simulink model "TestKit2"  (R2024b)
settings: Solver=FixedStepAuto  StartTime=0.0  StopTime=inf  FixedStep=0.1  RelTol=1e-3  EnableMultiTasking=on
libraries: stm32f4xxblockslib x8, stm32g4xxblockslib x6
settings Model: STM32="{\"EncoderBlockForG4\":[{\"ID\":\"TestKit2:1\"},{\"ID\":\"TestKit2:5\"},{\"ID\":\"TestKit2:7\"},{\"ID\":\"TestKit2:156\"},{\"ID\":\"TestKit2:157\"},{\"ID\":\"TestKit2:158\"}],\"DigitalPortRead\":[{\"ID\":\"TestKit2:112\"},{\"ID\":\"TestKit2:64\"},{\"ID\":\"TestKit2:65\"},{\"ID\":\"TestKit2:111\"},{\"ID\":\"TestKit2:128\"},{\"ID\":\"TestKit2:129\"},{\"ID\":\"TestKit2:130\"},{\"ID\":\"TestKit2:131\"}]}"  SimulationMode=external  Creator=KritZ  LastModifiedBy=KritZ
settings OptimizationCC: DefaultParameterBehavior=Inlined  EnhancedBackFolding=on  PassReuseOutputArgsAs=Individual arguments  ZeroExternalMemoryAtStartup=off  ZeroInternalMemoryAtStartup=off  MaxStackSize=512  OptimizeBlockOrder=speed  DifferentSizesBufferReuse=on  OptimizationCustomize=off  EfficientTunableParamExpr=on
settings DebuggingCC: ParameterTunabilityLossMsg=error
settings HardwareCC: ProdBitPerPointer=32  ProdBitPerSizeT=32  ProdBitPerPtrDiffT=32  ProdLargestAtomicInteger=Long  ProdLargestAtomicFloat=Double  ProdWordSize=32  ProdLongLongMode=on  ProdHWDeviceType=ARM Compatible->ARM Cortex-M
settings SFSimCC: MATLABDynamicMemAlloc=off
settings RTWCC: Description=Embedded Coder  SystemTargetFile=ert.tlc  HardwareBoard=STM32G4xx Based  TemplateMakefile=ert_default_tmf  Toolchain=GNU Tools for ARM Embedded Processors
settings CodeAppCC: ForceParamTrailComments=on  IgnoreCustomStorageClasses=off  OperatorAnnotations=on  SimulinkDataObjDesc=on  SFDataObjDesc=on  InsertBlockDesc=on
settings ERTTargetCC: TargetLangStandard=C99 (ISO)  CodeReplacementLibrary=ARM Cortex-M  SupportContinuousTime=on  ExtModeTransport=3  ExtModeStaticAlloc=on  ExtModeStaticAllocSize=2048  ExtModeMexFile=ext_xcp  ExtModeIntrfLevel=Level2 - Open

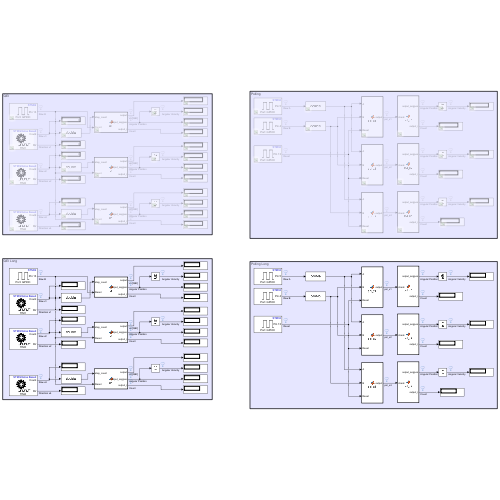
[thumbnail: Simulink's stored preview of the top-level diagram]
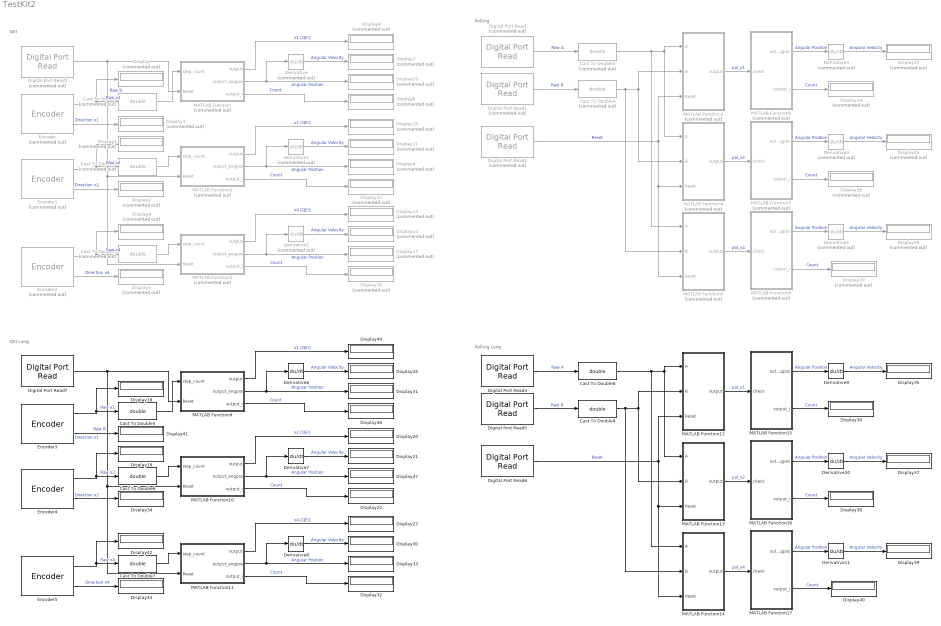
== system TestKit2 ==
  note: Polling
  note: QEI
  note: QEI Long
  note: Polling Long
  Cast To Double{,1..4} (5 alike) : DataTypeConversion  Commented=on  OutDataTypeStr=double  SaturateOnIntegerOverflow=off  RndMeth=Floor
  Cast To Double{5..9} (5 alike) : DataTypeConversion  OutDataTypeStr=double  SaturateOnIntegerOverflow=off  RndMeth=Floor
  Derivative{,1..5} (6 alike) : Derivative  Commented=on
  Derivative{6..11} (6 alike) : Derivative
  Digital Port Read : stm32f4xxblockslib/Digital Port Read  Commented=on  PortName=GPIOC  PinNumber=5  ReadOperation=on  IOAsArray=off  SampleTime=-1  EnableSimPort=off  hoistedMaskSrc=ECSoC/ECSimCodegen/Digital Port Read
      settings: LibrarySourceBlock=stm32g4xxblockslib/Digital Port Read
  Digital Port Read1 : stm32f4xxblockslib/Digital Port Read  Commented=on  PortName=GPIOC  PinNumber=4  ReadOperation=on  IOAsArray=off  SampleTime=-1  EnableSimPort=off  hoistedMaskSrc=ECSoC/ECSimCodegen/Digital Port Read
      settings: LibrarySourceBlock=stm32g4xxblockslib/Digital Port Read
  Digital Port Read2 : stm32f4xxblockslib/Digital Port Read  Commented=on  PortName=GPIOC  PinNumber=13  ReadOperation=on  IOAsArray=off  SampleTime=-1  EnableSimPort=off  hoistedMaskSrc=ECSoC/ECSimCodegen/Digital Port Read
      settings: LibrarySourceBlock=stm32g4xxblockslib/Digital Port Read
  Digital Port Read3 : stm32f4xxblockslib/Digital Port Read  Commented=on  PortName=GPIOC  PinNumber=13  ReadOperation=on  IOAsArray=off  SampleTime=-1  EnableSimPort=off  hoistedMaskSrc=ECSoC/ECSimCodegen/Digital Port Read
      settings: LibrarySourceBlock=stm32g4xxblockslib/Digital Port Read
  Digital Port Read4 : stm32f4xxblockslib/Digital Port Read  PortName=GPIOC  PinNumber=5  ReadOperation=on  IOAsArray=off  SampleTime=-1  EnableSimPort=off  hoistedMaskSrc=ECSoC/ECSimCodegen/Digital Port Read
      settings: LibrarySourceBlock=stm32g4xxblockslib/Digital Port Read
  Digital Port Read5 : stm32f4xxblockslib/Digital Port Read  PortName=GPIOC  PinNumber=4  ReadOperation=on  IOAsArray=off  SampleTime=-1  EnableSimPort=off  hoistedMaskSrc=ECSoC/ECSimCodegen/Digital Port Read
      settings: LibrarySourceBlock=stm32g4xxblockslib/Digital Port Read
  Digital Port Read6 : stm32f4xxblockslib/Digital Port Read  PortName=GPIOC  PinNumber=13  ReadOperation=on  IOAsArray=off  SampleTime=-1  EnableSimPort=off  hoistedMaskSrc=ECSoC/ECSimCodegen/Digital Port Read
      settings: LibrarySourceBlock=stm32g4xxblockslib/Digital Port Read
  Digital Port Read7 : stm32f4xxblockslib/Digital Port Read  PortName=GPIOC  PinNumber=13  ReadOperation=on  IOAsArray=off  SampleTime=-1  EnableSimPort=off  hoistedMaskSrc=ECSoC/ECSimCodegen/Digital Port Read
      settings: LibrarySourceBlock=stm32g4xxblockslib/Digital Port Read
  Display{,1..17,23..26,28..29} (24 alike) : Display  Commented=on
  Display{18..22,27,30..47} (24 alike) : Display
  Encoder : stm32g4xxblockslib/Encoder  Commented=on  TimerModule=TIM1  EnableResetInput=off  OutputCountAfterFirstIndex=off  OutputValidIndex=off  OutputDirection=on  OutputStatus=off  SampleTime=-1
  Encoder1 : stm32g4xxblockslib/Encoder  Commented=on  TimerModule=TIM3  EnableResetInput=off  OutputCountAfterFirstIndex=off  OutputValidIndex=off  OutputDirection=on  OutputStatus=off  SampleTime=-1
  Encoder2 : stm32g4xxblockslib/Encoder  Commented=on  TimerModule=TIM4  EnableResetInput=off  OutputCountAfterFirstIndex=off  OutputValidIndex=off  OutputDirection=on  OutputStatus=off  SampleTime=-1
  Encoder3 : stm32g4xxblockslib/Encoder  TimerModule=TIM1  EnableResetInput=off  OutputCountAfterFirstIndex=off  OutputValidIndex=off  OutputDirection=on  OutputStatus=off  SampleTime=-1
  Encoder4 : stm32g4xxblockslib/Encoder  TimerModule=TIM3  EnableResetInput=off  OutputCountAfterFirstIndex=off  OutputValidIndex=off  OutputDirection=on  OutputStatus=off  SampleTime=-1
  Encoder5 : stm32g4xxblockslib/Encoder  TimerModule=TIM4  EnableResetInput=off  OutputCountAfterFirstIndex=off  OutputValidIndex=off  OutputDirection=on  OutputStatus=off  SampleTime=-1
  MATLAB Function : MATLAB Function  Commented=on  TreatAsAtomicUnit=on
  MATLAB Function1 : MATLAB Function  Commented=on  TreatAsAtomicUnit=on
  MATLAB Function10 : MATLAB Function  TreatAsAtomicUnit=on
  MATLAB Function11 : MATLAB Function  TreatAsAtomicUnit=on
  MATLAB Function12 : MATLAB Function  TreatAsAtomicUnit=on
  MATLAB Function13 : MATLAB Function  TreatAsAtomicUnit=on
  MATLAB Function14 : MATLAB Function  TreatAsAtomicUnit=on
  MATLAB Function15 : MATLAB Function  TreatAsAtomicUnit=on
  MATLAB Function16 : MATLAB Function  TreatAsAtomicUnit=on
  MATLAB Function17 : MATLAB Function  TreatAsAtomicUnit=on
  MATLAB Function2 : MATLAB Function  Commented=on  TreatAsAtomicUnit=on
  MATLAB Function3 : MATLAB Function  Commented=on  TreatAsAtomicUnit=on
  MATLAB Function4 : MATLAB Function  Commented=on  TreatAsAtomicUnit=on
  MATLAB Function5 : MATLAB Function  Commented=on  TreatAsAtomicUnit=on
  MATLAB Function6 : MATLAB Function  Commented=on  TreatAsAtomicUnit=on
  MATLAB Function7 : MATLAB Function  Commented=on  TreatAsAtomicUnit=on
  MATLAB Function8 : MATLAB Function  Commented=on  TreatAsAtomicUnit=on
  MATLAB Function9 : MATLAB Function  TreatAsAtomicUnit=on
  wires:
  Encoder/1 -> Display/1, Cast To Double/1  "Raw x1"
  Encoder/2 -> Display3/1  "Direction x1"
  Encoder1/2 -> Display2/1  "Direction x2"
  Encoder1/1 -> Display1/1, Cast To Double1/1  "Raw x2"
  Encoder2/1 -> Display4/1, Cast To Double2/1  "Raw x4"
  Encoder2/2 -> Display5/1  "Direction x4"
  Cast To Double/1 -> MATLAB Function/1(step_count)
  MATLAB Function/1(output) -> Display6/1  "x1 [QEI]"
  MATLAB Function/3(output_i) -> Display8/1  "Count"
  MATLAB Function/2(output_angpos) -> Display15/1, Derivative/1  "Angular Position"
  Digital Port Read/1 -> Cast To Double3/1  "Raw A"
  Digital Port Read1/1 -> Cast To Double4/1  "Raw B"
  Cast To Double3/1 -> MATLAB Function5/1(A), MATLAB Function4/1(A), MATLAB Function3/1(A)
  Cast To Double4/1 -> MATLAB Function5/2(B), MATLAB Function3/2(B), MATLAB Function4/2(B)
  MATLAB Function3/1(output) -> MATLAB Function6/1(check)  "pol_x1"
  MATLAB Function5/1(output) -> MATLAB Function8/1(check)  "pol_x4"
  Derivative/1 -> Display7/1  "Angular Velocity"
  Derivative1/1 -> Display11/1  "Angular Velocity"
  MATLAB Function1/2(output_angpos) -> Display9/1, Derivative1/1  "Angular Position"
  MATLAB Function1/3(output_i) -> Display12/1  "Count"
  MATLAB Function1/1(output) -> Display10/1  "x2 [QEI]"
  Cast To Double1/1 -> MATLAB Function1/1(step_count)
  MATLAB Function2/2(output_angpos) -> Display17/1, Derivative2/1  "Angular Position"
  MATLAB Function2/1(output) -> Display13/1  "x4 [QEI]"
  MATLAB Function2/3(output_i) -> Display16/1  "Count"
  Derivative2/1 -> Display14/1  "Angular Velocity"
  Cast To Double2/1 -> MATLAB Function2/1(step_count)
  MATLAB Function6/1(output_angpos) -> Derivative3/1  "Angular Position"
  Derivative3/1 -> Display23/1  "Angular Velocity"
  MATLAB Function6/2(output_i) -> Display24/1  "Count"
  MATLAB Function4/1(output) -> MATLAB Function7/1(check)  "pol_x2"
  MATLAB Function7/1(output_angpos) -> Derivative4/1  "Angular Position"
  Derivative4/1 -> Display25/1  "Angular Velocity"
  MATLAB Function8/1(output_angpos) -> Derivative5/1  "Angular Position"
  Derivative5/1 -> Display28/1  "Angular Velocity"
  MATLAB Function8/2(output_i) -> Display29/1  "Count"
  MATLAB Function7/2(output_i) -> Display26/1  "Count"
  Digital Port Read2/1 -> MATLAB Function5/3(Reset), MATLAB Function4/3(Reset), MATLAB Function3/3(Reset)  "Reset"
  Digital Port Read3/1 -> MATLAB Function2/2(Reset), MATLAB Function1/2(Reset), MATLAB Function/2(Reset)  "Raw B"
  Digital Port Read5/1 -> Cast To Double9/1  "Raw B"
  Derivative11/1 -> Display39/1  "Angular Velocity"
  Digital Port Read7/1 -> MATLAB Function11/2(Reset), MATLAB Function10/2(Reset), MATLAB Function9/2(Reset)  "Raw B"
  Encoder5/2 -> Display43/1  "Direction x4"
  Digital Port Read4/1 -> Cast To Double8/1  "Raw A"
  MATLAB Function16/1(output_angpos) -> Derivative10/1  "Angular Position"
  Encoder5/1 -> Display42/1, Cast To Double7/1  "Raw x4"
  Derivative9/1 -> Display35/1  "Angular Velocity"
  Cast To Double9/1 -> MATLAB Function14/2(B), MATLAB Function12/2(B), MATLAB Function13/2(B)
  Cast To Double8/1 -> MATLAB Function14/1(A), MATLAB Function13/1(A), MATLAB Function12/1(A)
  Cast To Double6/1 -> MATLAB Function10/1(step_count)
  MATLAB Function11/3(output_i) -> Display32/1  "Count"
  MATLAB Function17/2(output_i) -> Display40/1  "Count"
  Encoder3/2 -> Display41/1  "Direction x1"
  MATLAB Function9/3(output_i) -> Display46/1  "Count"
  MATLAB Function12/1(output) -> MATLAB Function15/1(check)  "pol_x1"
  Encoder3/1 -> Display18/1, Cast To Double5/1  "Raw x1"
  MATLAB Function14/1(output) -> MATLAB Function17/1(check)  "pol_x4"
  MATLAB Function16/2(output_i) -> Display38/1  "Count"
  Derivative6/1 -> Display45/1  "Angular Velocity"
  MATLAB Function11/2(output_angpos) -> Display33/1, Derivative8/1  "Angular Position"
  Cast To Double7/1 -> MATLAB Function11/1(step_count)
  MATLAB Function15/1(output_angpos) -> Derivative9/1  "Angular Position"
  MATLAB Function9/2(output_angpos) -> Display31/1, Derivative6/1  "Angular Position"
  Digital Port Read6/1 -> MATLAB Function14/3(Reset), MATLAB Function13/3(Reset), MATLAB Function12/3(Reset)  "Reset"
  MATLAB Function11/1(output) -> Display27/1  "x4 [QEI]"
  MATLAB Function10/3(output_i) -> Display22/1  "Count"
  MATLAB Function10/2(output_angpos) -> Display47/1, Derivative7/1  "Angular Position"
  MATLAB Function13/1(output) -> MATLAB Function16/1(check)  "pol_x2"
  Derivative10/1 -> Display37/1  "Angular Velocity"
  MATLAB Function17/1(output_angpos) -> Derivative11/1  "Angular Position"
  Derivative7/1 -> Display21/1  "Angular Velocity"
  Encoder4/1 -> Display19/1, Cast To Double6/1  "Raw x2"
  MATLAB Function15/2(output_i) -> Display36/1  "Count"
  MATLAB Function10/1(output) -> Display20/1  "x2 [QEI]"
  Encoder4/2 -> Display34/1  "Direction x2"
  Cast To Double5/1 -> MATLAB Function9/1(step_count)
  MATLAB Function9/1(output) -> Display44/1  "x1 [QEI]"
  Derivative8/1 -> Display30/1  "Angular Velocity"

== matlab function TestKit2/MATLAB Function11 ==
  data: output output; step_count input; output_angpos output; output_i output; Reset input
function [output,output_angpos,output_i] = x4(step_count,Reset)
    % Local variebles
    persistent check;
    persistent previous;
    persistent rev;
    persistent degree;


    % Check the reset button
    if Reset == 1
        check = 0;
    end
   

    % Initialize the state
    if isempty(check)
        check = 0; 
    end
    if isempty(previous)
        previous = 0;
    end
    if isempty(rev)
        rev = 0;
    end
    if isempty(degree)
        degree = 0;
    end

    % Distance between an old and a new one (to create a unlimit graph)
    getnumber = step_count - previous;
    if getnumber < -32760
        check = (check + (65520 + getnumber))+1;
    elseif getnumber > 32760
        check = (check - (65520 - getnumber))-1;
    else 
        check = check + getnumber;
    end

                                                                                            
    % Get a last data to print out
    previous = step_count;
    

    % Revolute & Degree
    rev = check / 2048;
    degree = rev*360;


    % Show a step time, velocity, unlimitted for encoder in rotate
    output = check;
    output_angpos = degree;
    output_i = rev; 
end


% function [output,output_angvelo,output_angpos,output_i] = x1(step_count)
%     % Local variebles
%     persistent next; 
%     persistent previous;
%     persistent i;
% 
% 
%     % Initialize the state
%     if isempty(next)
%         next = 0; 
%     end
%     if isempty(previous)
%         previous = 0;
%     end
%     if isempty(i)
%         i = 0;
%     end
% 
% 
%     % Distance between an old and a new one (to create a unlimit graph)
%     getnumber = step_count-previous;
%     if getnumber <= -32760
%         getnumber = 1;
%     elseif getnumber >= 32760
%         getnumber = -1;
%     end
% 
% 
%     % Get a last data to print out
%     next = getnumber+next;
%     previous = step_count;
% 
% 
%     % Angular & Velocity
%     velocity = getnumber/0.1;
%     omeaga = velocity/9.5;
% 
% 
%     % Zeta & Radians
%     zeta = omeaga * 0.1;
%     radian = (pi/180)*zeta;
% 
% 
%     % Show a step time, velocity, unlimitted for encoder in rotate
%     output = next;
%     output_angvelo = omeaga;
%     output_angpos = radian;
%     output_i = floor(abs(next/24)); 
% end
% 
% function [output,output_angvelo,output_angpos,output_i] = x1(step_count)
%     % Local variebles
%     persistent check;
%     persistent previous;
%     persistent i;
% 
% 
%     % Initialize the state
%     if isempty(check)
%         check = 0; 
%     end
%     if isempty(previous)
%         previous = 0;
%     end
%     if isempty(i)
%         i = 0;
%     end
% 
% 
%     % Distance between an old and a new one (to create a unlimit graph)
%     getnumber = step_count-previous;
%     if getnumber < -32760
%         check = (check - (65520-getnumber))+1;
%     elseif getnumber > 32760
%         check = (check - (65520+getnumber))-1;
%     else 
%         check = check+getnumber;
%     end
% 
% 
%     % Get a last data to print out
%     previous = step_count;
% 
% 
%     % Angular & Velocity
%     velocity = getnumber/0.1;
%     omeaga = velocity/9.5;
% 
% 
%     % Zeta & Radians
%     zeta = omeaga * 0.1;
%     radian = (pi/180)*zeta;
% 
% 
%     % Show a step time, velocity, unlimitted for encoder in rotate
%     output = check;
%     output_angvelo = omeaga;
%     output_angpos = radian;
%     output_i = floor(abs(check/24)); 
% end

== matlab function TestKit2/MATLAB Function12 ==
  data: A input; output output; B input; Reset input
function output = pol_x1(A,B,Reset)
    % Identifly a variable
    persistent count; 
    persistent previous;
    

    % Check the reset button
    if Reset == 1
        count = 0;
    end

    
    % Initialize the state on the first call
    if isempty(count)
        count = 0;
    end
    if isempty(previous)
        previous = 0;
    end
    

    % Condition for x1 [clockwise and counter-clockwise]
    if A == 1 && previous == 0
        if A == 1 && B == 0
            count = count + 1;
        elseif A == 1 && B == 1
            count = count - 1;
        end
    end


    % Get a last data to print out
    previous = A;


    % Output
    output = count;

== matlab function TestKit2/MATLAB Function1 ==
  data: output output; step_count input; output_angpos output; output_i output; Reset input
function [output,output_angpos,output_i] = x2(step_count,Reset)
    % Local variebles
    persistent check;
    persistent previous;
    persistent rev;
    persistent degree;


    % Check the reset button
    if Reset == 1
        check = 0;
    end
   

    % Initialize the state
    if isempty(check)
        check = 0; 
    end
    if isempty(previous)
        previous = 0;
    end
    if isempty(rev)
        rev = 0;
    end
    if isempty(degree)
        degree = 0;
    end

    % Distance between an old and a new one (to create a unlimit graph)
    getnumber = step_count - previous;
    if getnumber < -32760
        check = (check + (65520 + getnumber))+1;
    elseif getnumber > 32760
        check = (check - (65520 - getnumber))-1;
    else 
        check = check + getnumber;
    end

                                                                                            
    % Get a last data to print out
    previous = step_count;
    

    % Revolute & Degree
    rev = check / 24;
    degree = rev*360;


    % Show a step time, velocity, unlimitted for encoder in rotate
    output = check;
    output_angpos = degree;
    output_i = rev; 
end


% function [output,output_angvelo,output_angpos,output_i] = x1(step_count)
%     % Local variebles
%     persistent next; 
%     persistent previous;
%     persistent i;
% 
% 
%     % Initialize the state
%     if isempty(next)
%         next = 0; 
%     end
%     if isempty(previous)
%         previous = 0;
%     end
%     if isempty(i)
%         i = 0;
%     end
% 
% 
%     % Distance between an old and a new one (to create a unlimit graph)
%     getnumber = step_count-previous;
%     if getnumber <= -32760
%         getnumber = 1;
%     elseif getnumber >= 32760
%         getnumber = -1;
%     end
% 
% 
%     % Get a last data to print out
%     next = getnumber+next;
%     previous = step_count;
% 
% 
%     % Angular & Velocity
%     velocity = getnumber/0.1;
%     omeaga = velocity/9.5;
% 
% 
%     % Zeta & Radians
%     zeta = omeaga * 0.1;
%     radian = (pi/180)*zeta;
% 
% 
%     % Show a step time, velocity, unlimitted for encoder in rotate
%     output = next;
%     output_angvelo = omeaga;
%     output_angpos = radian;
%     output_i = floor(abs(next/24)); 
% end
% 
% function [output,output_angvelo,output_angpos,output_i] = x1(step_count)
%     % Local variebles
%     persistent check;
%     persistent previous;
%     persistent i;
% 
% 
%     % Initialize the state
%     if isempty(check)
%         check = 0; 
%     end
%     if isempty(previous)
%         previous = 0;
%     end
%     if isempty(i)
%         i = 0;
%     end
% 
% 
%     % Distance between an old and a new one (to create a unlimit graph)
%     getnumber = step_count-previous;
%     if getnumber < -32760
%         check = (check - (65520-getnumber))+1;
%     elseif getnumber > 32760
%         check = (check - (65520+getnumber))-1;
%     else 
%         check = check+getnumber;
%     end
% 
% 
%     % Get a last data to print out
%     previous = step_count;
% 
% 
%     % Angular & Velocity
%     velocity = getnumber/0.1;
%     omeaga = velocity/9.5;
% 
% 
%     % Zeta & Radians
%     zeta = omeaga * 0.1;
%     radian = (pi/180)*zeta;
% 
% 
%     % Show a step time, velocity, unlimitted for encoder in rotate
%     output = check;
%     output_angvelo = omeaga;
%     output_angpos = radian;
%     output_i = floor(abs(check/24)); 
% end

== matlab function TestKit2/MATLAB Function13 ==
  data: A input; output output; B input; Reset input
function output = pol_x2(A,B,Reset)
    % Identifly a variable
    persistent count; 
    persistent previous;
    

    % Check the reset button
    if Reset == 1
        count = 0;
    end


    % Initialize the state on the first call
    if isempty(count)
        count = 0;
    end
    if isempty(previous)
        previous = 0;
    end
    

    % Condition for x2 [clockwise and counter-clockwise]
    if A == 1 && previous == 0
        if A == 1 && B == 0
            count = count + 1;
        elseif A == 0 && B == 1
            count = count + 1;
        elseif A == 1 && B == 1
            count = count - 1;
        elseif A == 0 && B == 0
            count = count - 1;
        end 
    elseif A == 0 && previous == 1
        if A == 1 && B == 0
            count = count + 1;
        elseif A == 0 && B == 1
            count = count + 1;
        elseif A == 1 && B == 1
            count = count - 1;
        elseif A == 0 && B == 0
            count = count - 1;
        end  
    end


    % Get a last data to print out
    previous = A;


    % Output
    output = count;

== matlab function TestKit2/MATLAB Function14 ==
  data: A input; output output; B input; Reset input
function output = pol_x4(A,B,Reset)
    % Identifly a variable
    persistent count; 
    persistent previous_A;
    persistent previous_B;


    % Check the reset button
    if Reset == 1
        count = 0;
    end


    % Initialize the state on the first call
    if isempty(count)
        count = 0;
    end
    if isempty(previous_A)
        previous_A = 0;
    end
    if isempty(previous_B)
        previous_B = 0;
    end


    % Condition for x4A & x4B [clockwise and counter-clockwise]
    if A == 1 && previous_A == 0
        if B == 0
            count = count + 1;
        else 
            count = count - 1;
        end
    elseif A == 0 && previous_A == 1 
        if B == 1
            count = count + 1;
        else 
            count = count - 1;
        end
    elseif B == 1 && previous_B == 0
        if A == 1
            count = count + 1;
        else 
            count = count - 1;
        end
    elseif B == 0 && previous_B == 1 
        if A == 0
            count = count + 1;
        else
            count = count - 1;
        end
    end


    % Get a last data to print out
    previous_A = A;
    previous_B = B;


    % Output
    output = count;

== matlab function TestKit2/MATLAB Function15 ==
  data: check input; output_angpos output; output_i output
function [output_angpos,output_i] = out_x1(check)
    % Identifly a variable
    persistent count;


    % Initialize the state on the first call
    if isempty(count)
        count = 0;
    end


    % Revolute & Degree
    rev = check / 2048;
    degree = rev*360;
    radian = degree*2*pi;


    % Show a step time, velocity for encoder in rotate
    output_angpos = radian;
    output_i = rev;

== matlab function TestKit2/MATLAB Function16 ==
  data: check input; output_angpos output; output_i output
function [output_angpos,output_i] = out_x2(check)
    % Identifly a variable
    persistent count;


    % Initialize the state on the first call
    if isempty(count)
        count = 0;
    end


    % Revolute & Degree
    rev = check / (2048*2);
    degree = rev*360;
    radian = degree*2*pi;


    % Show a step time, velocity for encoder in rotate
    output_angpos = radian;
    output_i = rev;

== matlab function TestKit2/MATLAB Function17 ==
  data: check input; output_angpos output; output_i output
function [output_angpos,output_i] = out_x4(check)
    % Identifly a variable
    persistent count;


    % Initialize the state on the first call
    if isempty(count)
        count = 0;
    end


    % Revolute & Degree
    rev = check / (2048*4);
    degree = rev*360;
    radian = degree*2*pi;


    % Show a step time, velocity for encoder in rotate
    output_angpos = radian;
    output_i = rev;

== matlab function TestKit2/MATLAB Function9 ==
  data: output output; step_count input; output_angpos output; output_i output; Reset input
function [output,output_angpos,output_i] = x1(step_count,Reset)
    % Local variebles
    persistent check;
    persistent previous;
    persistent rev;
    persistent degree;


    % Check the reset button
    if Reset == 1
        check = 0;
    end
   

    % Initialize the state
    if isempty(check)
        check = 0; 
    end
    if isempty(previous)
        previous = 0;
    end
    if isempty(rev)
        rev = 0;
    end
    if isempty(degree)
        degree = 0;
    end

    % Distance between an old and a new one (to create a unlimit graph)
    getnumber = step_count - previous;
    if getnumber < -32760
        check = (check + (65520 + getnumber))+1;
    elseif getnumber > 32760
        check = (check - (65520 - getnumber))-1;
    else 
        check = check + getnumber;
    end

                                                                                            
    % Get a last data to print out
    previous = step_count;
    

    % Revolute & Degree
    rev = check / 2048;
    degree = rev*360;


    % Show a step time, velocity, unlimitted for encoder in rotate
    output = check;
    output_angpos = degree;
    output_i = rev; 
end


% function [output,output_angvelo,output_angpos,output_i] = x1(step_count)
%     % Local variebles
%     persistent next; 
%     persistent previous;
%     persistent i;
% 
% 
%     % Initialize the state
%     if isempty(next)
%         next = 0; 
%     end
%     if isempty(previous)
%         previous = 0;
%     end
%     if isempty(i)
%         i = 0;
%     end
% 
% 
%     % Distance between an old and a new one (to create a unlimit graph)
%     getnumber = step_count-previous;
%     if getnumber <= -32760
%         getnumber = 1;
%     elseif getnumber >= 32760
%         getnumber = -1;
%     end
% 
% 
%     % Get a last data to print out
%     next = getnumber+next;
%     previous = step_count;
% 
% 
%     % Angular & Velocity
%     velocity = getnumber/0.1;
%     omeaga = velocity/9.5;
% 
% 
%     % Zeta & Radians
%     zeta = omeaga * 0.1;
%     radian = (pi/180)*zeta;
% 
% 
%     % Show a step time, velocity, unlimitted for encoder in rotate
%     output = next;
%     output_angvelo = omeaga;
%     output_angpos = radian;
%     output_i = floor(abs(next/24)); 
% end
% 
% function [output,output_angvelo,output_angpos,output_i] = x1(step_count)
%     % Local variebles
%     persistent check;
%     persistent previous;
%     persistent i;
% 
% 
%     % Initialize the state
%     if isempty(check)
%         check = 0; 
%     end
%     if isempty(previous)
%         previous = 0;
%     end
%     if isempty(i)
%         i = 0;
%     end
% 
% 
%     % Distance between an old and a new one (to create a unlimit graph)
%     getnumber = step_count-previous;
%     if getnumber < -32760
%         check = (check - (65520-getnumber))+1;
%     elseif getnumber > 32760
%         check = (check - (65520+getnumber))-1;
%     else 
%         check = check+getnumber;
%     end
% 
% 
%     % Get a last data to print out
%     previous = step_count;
% 
% 
%     % Angular & Velocity
%     velocity = getnumber/0.1;
%     omeaga = velocity/9.5;
% 
% 
%     % Zeta & Radians
%     zeta = omeaga * 0.1;
%     radian = (pi/180)*zeta;
% 
% 
%     % Show a step time, velocity, unlimitted for encoder in rotate
%     output = check;
%     output_angvelo = omeaga;
%     output_angpos = radian;
%     output_i = floor(abs(check/24)); 
% end

== matlab function TestKit2/MATLAB Function ==
  data: output output; step_count input; output_angpos output; output_i output; Reset input
function [output,output_angpos,output_i] = x1(step_count,Reset)
    % Local variebles
    persistent check;
    persistent previous;
    persistent rev;
    persistent degree;


    % Check the reset button
    if Reset == 1
        check = 0;
    end
   

    % Initialize the state
    if isempty(check)
        check = 0; 
    end
    if isempty(previous)
        previous = 0;
    end
    if isempty(rev)
        rev = 0;
    end
    if isempty(degree)
        degree = 0;
    end

    % Distance between an old and a new one (to create a unlimit graph)
    getnumber = step_count - previous;
    if getnumber < -32760
        check = (check + (65520 + getnumber))+1;
    elseif getnumber > 32760
        check = (check - (65520 - getnumber))-1;
    else 
        check = check + getnumber;
    end

                                                                                            
    % Get a last data to print out
    previous = step_count;
    

    % Revolute & Degree
    rev = check / 24;
    degree = rev*360;


    % Show a step time, velocity, unlimitted for encoder in rotate
    output = check;
    output_angpos = degree;
    output_i = rev; 
end


% function [output,output_angvelo,output_angpos,output_i] = x1(step_count)
%     % Local variebles
%     persistent next; 
%     persistent previous;
%     persistent i;
% 
% 
%     % Initialize the state
%     if isempty(next)
%         next = 0; 
%     end
%     if isempty(previous)
%         previous = 0;
%     end
%     if isempty(i)
%         i = 0;
%     end
% 
% 
%     % Distance between an old and a new one (to create a unlimit graph)
%     getnumber = step_count-previous;
%     if getnumber <= -32760
%         getnumber = 1;
%     elseif getnumber >= 32760
%         getnumber = -1;
%     end
% 
% 
%     % Get a last data to print out
%     next = getnumber+next;
%     previous = step_count;
% 
% 
%     % Angular & Velocity
%     velocity = getnumber/0.1;
%     omeaga = velocity/9.5;
% 
% 
%     % Zeta & Radians
%     zeta = omeaga * 0.1;
%     radian = (pi/180)*zeta;
% 
% 
%     % Show a step time, velocity, unlimitted for encoder in rotate
%     output = next;
%     output_angvelo = omeaga;
%     output_angpos = radian;
%     output_i = floor(abs(next/24)); 
% end
% 
% function [output,output_angvelo,output_angpos,output_i] = x1(step_count)
%     % Local variebles
%     persistent check;
%     persistent previous;
%     persistent i;
% 
% 
%     % Initialize the state
%     if isempty(check)
%         check = 0; 
%     end
%     if isempty(previous)
%         previous = 0;
%     end
%     if isempty(i)
%         i = 0;
%     end
% 
% 
%     % Distance between an old and a new one (to create a unlimit graph)
%     getnumber = step_count-previous;
%     if getnumber < -32760
%         check = (check - (65520-getnumber))+1;
%     elseif getnumber > 32760
%         check = (check - (65520+getnumber))-1;
%     else 
%         check = check+getnumber;
%     end
% 
% 
%     % Get a last data to print out
%     previous = step_count;
% 
% 
%     % Angular & Velocity
%     velocity = getnumber/0.1;
%     omeaga = velocity/9.5;
% 
% 
%     % Zeta & Radians
%     zeta = omeaga * 0.1;
%     radian = (pi/180)*zeta;
% 
% 
%     % Show a step time, velocity, unlimitted for encoder in rotate
%     output = check;
%     output_angvelo = omeaga;
%     output_angpos = radian;
%     output_i = floor(abs(check/24)); 
% end

== matlab function TestKit2/MATLAB Function2 ==
  data: output output; step_count input; output_angpos output; output_i output; Reset input
function [output,output_angpos,output_i] = x4(step_count,Reset)
    % Local variebles
    persistent check;
    persistent previous;
    persistent rev;
    persistent degree;


    % Check the reset button
    if Reset == 1
        check = 0;
    end
   

    % Initialize the state
    if isempty(check)
        check = 0; 
    end
    if isempty(previous)
        previous = 0;
    end
    if isempty(rev)
        rev = 0;
    end
    if isempty(degree)
        degree = 0;
    end

    % Distance between an old and a new one (to create a unlimit graph)
    getnumber = step_count - previous;
    if getnumber < -32760
        check = (check + (65520 + getnumber))+1;
    elseif getnumber > 32760
        check = (check - (65520 - getnumber))-1;
    else 
        check = check + getnumber;
    end

                                                                                            
    % Get a last data to print out
    previous = step_count;
    

    % Revolute & Degree
    rev = check / 24;
    degree = rev*360;


    % Show a step time, velocity, unlimitted for encoder in rotate
    output = check;
    output_angpos = degree;
    output_i = rev; 
end


% function [output,output_angvelo,output_angpos,output_i] = x1(step_count)
%     % Local variebles
%     persistent next; 
%     persistent previous;
%     persistent i;
% 
% 
%     % Initialize the state
%     if isempty(next)
%         next = 0; 
%     end
%     if isempty(previous)
%         previous = 0;
%     end
%     if isempty(i)
%         i = 0;
%     end
% 
% 
%     % Distance between an old and a new one (to create a unlimit graph)
%     getnumber = step_count-previous;
%     if getnumber <= -32760
%         getnumber = 1;
%     elseif getnumber >= 32760
%         getnumber = -1;
%     end
% 
% 
%     % Get a last data to print out
%     next = getnumber+next;
%     previous = step_count;
% 
% 
%     % Angular & Velocity
%     velocity = getnumber/0.1;
%     omeaga = velocity/9.5;
% 
% 
%     % Zeta & Radians
%     zeta = omeaga * 0.1;
%     radian = (pi/180)*zeta;
% 
% 
%     % Show a step time, velocity, unlimitted for encoder in rotate
%     output = next;
%     output_angvelo = omeaga;
%     output_angpos = radian;
%     output_i = floor(abs(next/24)); 
% end
% 
% function [output,output_angvelo,output_angpos,output_i] = x1(step_count)
%     % Local variebles
%     persistent check;
%     persistent previous;
%     persistent i;
% 
% 
%     % Initialize the state
%     if isempty(check)
%         check = 0; 
%     end
%     if isempty(previous)
%         previous = 0;
%     end
%     if isempty(i)
%         i = 0;
%     end
% 
% 
%     % Distance between an old and a new one (to create a unlimit graph)
%     getnumber = step_count-previous;
%     if getnumber < -32760
%         check = (check - (65520-getnumber))+1;
%     elseif getnumber > 32760
%         check = (check - (65520+getnumber))-1;
%     else 
%         check = check+getnumber;
%     end
% 
% 
%     % Get a last data to print out
%     previous = step_count;
% 
% 
%     % Angular & Velocity
%     velocity = getnumber/0.1;
%     omeaga = velocity/9.5;
% 
% 
%     % Zeta & Radians
%     zeta = omeaga * 0.1;
%     radian = (pi/180)*zeta;
% 
% 
%     % Show a step time, velocity, unlimitted for encoder in rotate
%     output = check;
%     output_angvelo = omeaga;
%     output_angpos = radian;
%     output_i = floor(abs(check/24)); 
% end

== matlab function TestKit2/MATLAB Function3 ==
  data: A input; output output; B input; Reset input
function output = pol_x1(A,B,Reset)
    % Identifly a variable
    persistent count; 
    persistent previous;
    

    % Check the reset button
    if Reset == 1
        count = 0;
    end

    
    % Initialize the state on the first call
    if isempty(count)
        count = 0;
    end
    if isempty(previous)
        previous = 0;
    end
    

    % Condition for x1 [clockwise and counter-clockwise]
    if A == 1 && previous == 0
        if A == 1 && B == 0
            count = count + 1;
        elseif A == 1 && B == 1
            count = count - 1;
        end
    end


    % Get a last data to print out
    previous = A;


    % Output
    output = count;

== matlab function TestKit2/MATLAB Function4 ==
  data: A input; output output; B input; Reset input
function output = pol_x2(A,B,Reset)
    % Identifly a variable
    persistent count; 
    persistent previous;
    

    % Check the reset button
    if Reset == 1
        count = 0;
    end


    % Initialize the state on the first call
    if isempty(count)
        count = 0;
    end
    if isempty(previous)
        previous = 0;
    end
    

    % Condition for x2 [clockwise and counter-clockwise]
    if A == 1 && previous == 0
        if A == 1 && B == 0
            count = count + 1;
        elseif A == 0 && B == 1
            count = count + 1;
        elseif A == 1 && B == 1
            count = count - 1;
        elseif A == 0 && B == 0
            count = count - 1;
        end 
    elseif A == 0 && previous == 1
        if A == 1 && B == 0
            count = count + 1;
        elseif A == 0 && B == 1
            count = count + 1;
        elseif A == 1 && B == 1
            count = count - 1;
        elseif A == 0 && B == 0
            count = count - 1;
        end  
    end


    % Get a last data to print out
    previous = A;


    % Output
    output = count;

== matlab function TestKit2/MATLAB Function5 ==
  data: A input; output output; B input; Reset input
function output = pol_x4(A,B,Reset)
    % Identifly a variable
    persistent count; 
    persistent previous_A;
    persistent previous_B;


    % Check the reset button
    if Reset == 1
        count = 0;
    end


    % Initialize the state on the first call
    if isempty(count)
        count = 0;
    end
    if isempty(previous_A)
        previous_A = 0;
    end
    if isempty(previous_B)
        previous_B = 0;
    end


    % Condition for x4A & x4B [clockwise and counter-clockwise]
    if A == 1 && previous_A == 0
        if B == 0
            count = count + 1;
        else 
            count = count - 1;
        end
    elseif A == 0 && previous_A == 1 
        if B == 1
            count = count + 1;
        else 
            count = count - 1;
        end
    elseif B == 1 && previous_B == 0
        if A == 1
            count = count + 1;
        else 
            count = count - 1;
        end
    elseif B == 0 && previous_B == 1 
        if A == 0
            count = count + 1;
        else
            count = count - 1;
        end
    end


    % Get a last data to print out
    previous_A = A;
    previous_B = B;


    % Output
    output = count;

== matlab function TestKit2/MATLAB Function6 ==
  data: check input; output_angpos output; output_i output
function [output_angpos,output_i] = out_x1(check)
    % Identifly a variable
    persistent count;


    % Initialize the state on the first call
    if isempty(count)
        count = 0;
    end


    % Revolute & Degree
    rev = check / 24;
    degree = rev*360;
    radian = degree*2*pi;


    % Show a step time, velocity for encoder in rotate
    output_angpos = radian;
    output_i = rev;

== matlab function TestKit2/MATLAB Function7 ==
  data: check input; output_angpos output; output_i output
function [output_angpos,output_i] = out_x2(check)
    % Identifly a variable
    persistent count;


    % Initialize the state on the first call
    if isempty(count)
        count = 0;
    end


    % Revolute & Degree
    rev = check / 48;
    degree = rev*360;
    radian = degree*2*pi;


    % Show a step time, velocity for encoder in rotate
    output_angpos = radian;
    output_i = rev;

== matlab function TestKit2/MATLAB Function8 ==
  data: check input; output_angpos output; output_i output
function [output_angpos,output_i] = out_x4(check)
    % Identifly a variable
    persistent count;


    % Initialize the state on the first call
    if isempty(count)
        count = 0;
    end


    % Revolute & Degree
    rev = check / 96;
    degree = rev*360;
    radian = degree*2*pi;


    % Show a step time, velocity for encoder in rotate
    output_angpos = radian;
    output_i = rev;

== matlab function TestKit2/MATLAB Function10 ==
  data: output output; step_count input; output_angpos output; output_i output; Reset input
function [output,output_angpos,output_i] = x2(step_count,Reset)
    % Local variebles
    persistent check;
    persistent previous;
    persistent rev;
    persistent degree;


    % Check the reset button
    if Reset == 1
        check = 0;
    end
   

    % Initialize the state
    if isempty(check)
        check = 0; 
    end
    if isempty(previous)
        previous = 0;
    end
    if isempty(rev)
        rev = 0;
    end
    if isempty(degree)
        degree = 0;
    end

    % Distance between an old and a new one (to create a unlimit graph)
    getnumber = step_count - previous;
    if getnumber < -32760
        check = (check + (65520 + getnumber))+1;
    elseif getnumber > 32760
        check = (check - (65520 - getnumber))-1;
    else 
        check = check + getnumber;
    end

                                                                                            
    % Get a last data to print out
    previous = step_count;
    

    % Revolute & Degree
    rev = check / 2048;
    degree = rev*360;


    % Show a step time, velocity, unlimitted for encoder in rotate
    output = check;
    output_angpos = degree;
    output_i = rev; 
end


% function [output,output_angvelo,output_angpos,output_i] = x1(step_count)
%     % Local variebles
%     persistent next; 
%     persistent previous;
%     persistent i;
% 
% 
%     % Initialize the state
%     if isempty(next)
%         next = 0; 
%     end
%     if isempty(previous)
%         previous = 0;
%     end
%     if isempty(i)
%         i = 0;
%     end
% 
% 
%     % Distance between an old and a new one (to create a unlimit graph)
%     getnumber = step_count-previous;
%     if getnumber <= -32760
%         getnumber = 1;
%     elseif getnumber >= 32760
%         getnumber = -1;
%     end
% 
% 
%     % Get a last data to print out
%     next = getnumber+next;
%     previous = step_count;
% 
% 
%     % Angular & Velocity
%     velocity = getnumber/0.1;
%     omeaga = velocity/9.5;
% 
% 
%     % Zeta & Radians
%     zeta = omeaga * 0.1;
%     radian = (pi/180)*zeta;
% 
% 
%     % Show a step time, velocity, unlimitted for encoder in rotate
%     output = next;
%     output_angvelo = omeaga;
%     output_angpos = radian;
%     output_i = floor(abs(next/24)); 
% end
% 
% function [output,output_angvelo,output_angpos,output_i] = x1(step_count)
%     % Local variebles
%     persistent check;
%     persistent previous;
%     persistent i;
% 
% 
%     % Initialize the state
%     if isempty(check)
%         check = 0; 
%     end
%     if isempty(previous)
%         previous = 0;
%     end
%     if isempty(i)
%         i = 0;
%     end
% 
% 
%     % Distance between an old and a new one (to create a unlimit graph)
%     getnumber = step_count-previous;
%     if getnumber < -32760
%         check = (check - (65520-getnumber))+1;
%     elseif getnumber > 32760
%         check = (check - (65520+getnumber))-1;
%     else 
%         check = check+getnumber;
%     end
% 
% 
%     % Get a last data to print out
%     previous = step_count;
% 
% 
%     % Angular & Velocity
%     velocity = getnumber/0.1;
%     omeaga = velocity/9.5;
% 
% 
%     % Zeta & Radians
%     zeta = omeaga * 0.1;
%     radian = (pi/180)*zeta;
% 
% 
%     % Show a step time, velocity, unlimitted for encoder in rotate
%     output = check;
%     output_angvelo = omeaga;
%     output_angpos = radian;
%     output_i = floor(abs(check/24)); 
% end
